simulink library "lowFreqFlowData_ul"  (R2022a)
settings: Solver=VariableStepAuto  StartTime=0.0  StopTime=10.0  RelTol=1e-3
undefined symbols (not defined in the file or in its folder): env
settings Model: Creator=M.Cobb  LastModifiedBy=lhill8
settings SolverCC: AlgebraicLoopSolver=TrustRegion
settings DebuggingCC: UnconnectedInputMsg=warning  UnconnectedOutputMsg=warning  UnconnectedLineMsg=warning  SFMachineParentedDataDiag=warning  ArithmeticOperatorsInVariantConditions=warning
settings SFSimCC: CustomCodeUndefinedFunction=UseInterfaceOnly

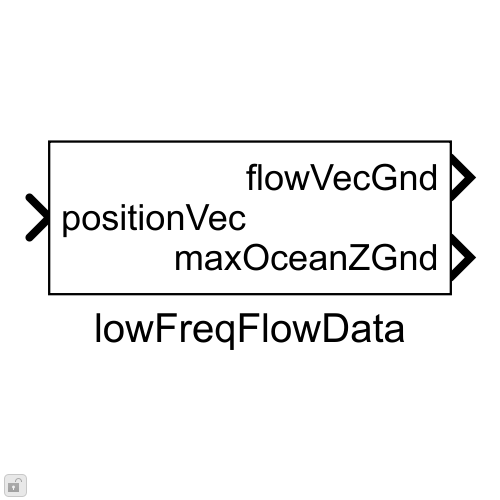
[thumbnail: Simulink's stored preview of the top-level diagram]
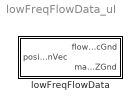
== system lowFreqFlowData_ul ==
  lowFreqFlowData : Subsystem  VariantControl=VSS_flowCalculation_constXYZT

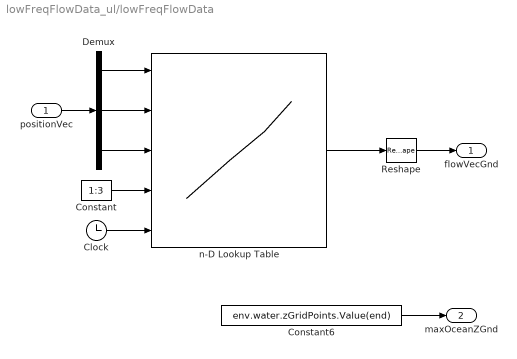
== system lowFreqFlowData_ul/lowFreqFlowData ==
  positionVec : Inport  PortDimensions=[3 1]
  Clock : Clock
  Constant : Constant  Value=1:3
  Constant6 : Constant  Value=env.water.zGridPoints.Value(end)
  Demux : Demux  Outputs=3
  Reshape : Reshape  OutputDimensionality=Column vector (2-D)
  n-D Lookup Table : Lookup_n-D  NumberOfTableDimensions=5  BreakpointsForDimension1=env.water.xGridPoints.Value  BreakpointsForDimension2=env.water.yGridPoints.Value  BreakpointsForDimension3=env.water.zGridPoints.Value  BreakpointsForDimension4=1:3  BreakpointsForDimension5=env.water.flowVecTimeseries.Value.Time  BeginIndexSearchUsingPreviousIndexResult=on  Table=env.water.flowVecTimeseries.Value.Data  ExtrapMethod=Clip  UseLastTableValue=on  InternalRulePriority=Speed  RndMeth=Simplest
      settings: InputPortMap=u0,u1,u2,u3,u4
  flowVecGnd : Outport  VectorParamsAs1DForOutWhenUnconnected=off
  maxOceanZGnd : Outport  Port=2  VectorParamsAs1DForOutWhenUnconnected=off
  wires:
  Demux/1 -> n-D Lookup Table/1
  Demux/2 -> n-D Lookup Table/2
  Demux/3 -> n-D Lookup Table/3
  positionVec/1 -> Demux/1
  n-D Lookup Table/1 -> Reshape/1
  Reshape/1 -> flowVecGnd/1
  Constant/1 -> n-D Lookup Table/4
  Clock/1 -> n-D Lookup Table/5
  Constant6/1 -> maxOceanZGnd/1
